simulink model "Lab1_Prelab"  (R2019a)
settings: Solver=VariableStepAuto  StartTime=0.0  StopTime=10.0  RelTol=1e-3
undefined symbols (not defined in the file or in its folder): G1, G2, K, s
settings Model: Creator=Gabe Casciano  LastModifiedBy=Gabe Casciano

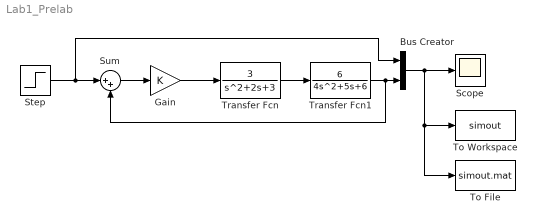
== system Lab1_Prelab ==
  Bus Creator : BusCreator  Inputs=2
  Gain : Gain  Gain=K
  Scope : Scope
  Step : Step  SampleTime=0
  Sum : Sum  Inputs=|++
  To File : ToFile  Filename=simout.mat  SaveFormat=Timeseries
  To Workspace : ToWorkspace  VariableName=simout  SaveFormat=Timeseries  SampleTime=-1
  Transfer Fcn : TransferFcn  Numerator=[3]  Denominator=[1 2 3]  ContinuousStateAttributes=G1(s)
  Transfer Fcn1 : TransferFcn  Numerator=[6]  Denominator=[4 5 6]  ContinuousStateAttributes=G2(s)
  wires:
  Sum/1 -> Gain/1
  Gain/1 -> Transfer Fcn/1
  Transfer Fcn/1 -> Transfer Fcn1/1
  Transfer Fcn1/1 -> Sum/2, Bus Creator/2
  Step/1 -> Sum/1, Bus Creator/1
  Bus Creator/1 -> To File/1, To Workspace/1, Scope/1
